simulink model "data_genrator"  (R2025b)
settings: Solver=FixedStepDiscrete  StartTime=0.0  StopTime=1800  FixedStep=2  RelTol=1e-3
libraries: instrumentseriallib x2
settings Model: Creator=Dell  LastModifiedBy=Dell

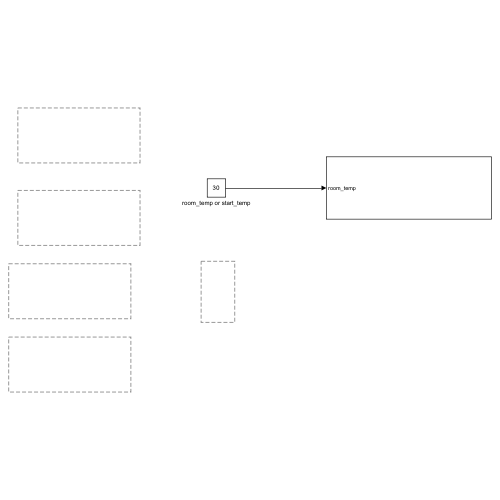
[thumbnail: Simulink's stored preview of the top-level diagram]
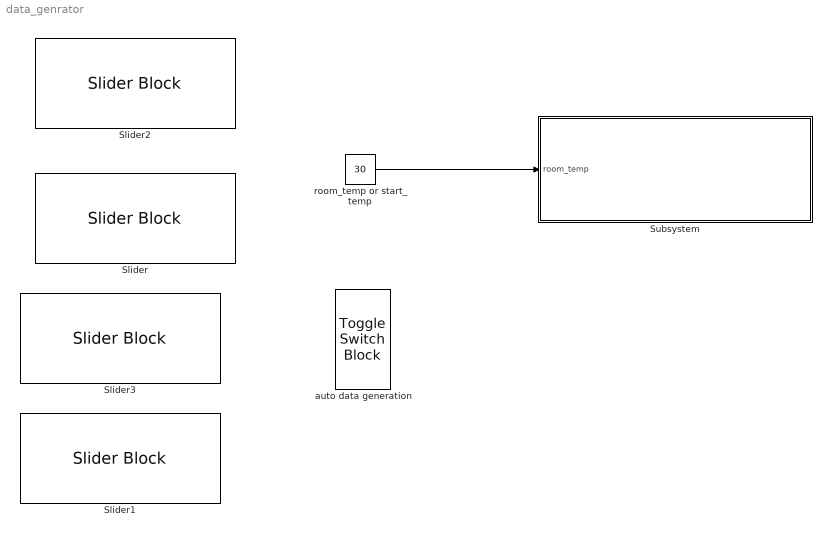
== system data_genrator ==
  Slider : SliderBlock
  Slider1 : SliderBlock  ScaleMax=2
  Slider2 : SliderBlock
  Slider3 : SliderBlock  ScaleMax=2
  Subsystem : Subsystem
  "auto data generation " : ToggleSwitchBlock
  room_temp or start_temp : Constant  Value=30
  wires:
  room_temp or start_temp/1 -> Subsystem/1(room_temp)

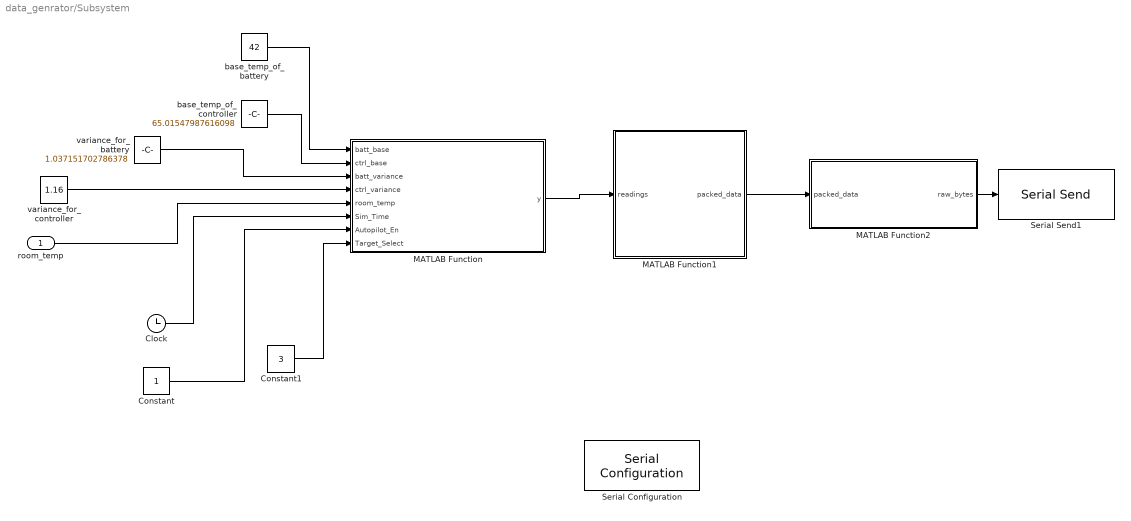
== system data_genrator/Subsystem ==
  room_temp : Inport
  Clock : Clock
  Constant : Constant
  Constant1 : Constant  Value=3
  MATLAB Function : MATLAB Function  TreatAsAtomicUnit=on
  MATLAB Function1 : MATLAB Function  TreatAsAtomicUnit=on
  MATLAB Function2 : MATLAB Function  TreatAsAtomicUnit=on
  Serial Configuration : instrumentseriallib/Serial Configuration  Priority=-200000  PortSel=COM8  Port=COM8  ComPort=COM8  BaudRate=115200  DataBits=8  Parity=none  StopBits=1  ByteOrder=little-endian  FlowControl=none  Timeout=10  SimulateUsing=Interpreted execution  BlockInModel=on  aMode=1
  Serial Send1 : instrumentseriallib/Serial Send  Priority=1  PortSel=COM8  Port=COM8  ComPort=COM8  Header=[]  Terminator=<none>  CustomTerminator=[]  EnableBlockingMode=on  SimulateUsing=Interpreted execution  BlockInModel=on  aMode=1
  base_temp_of_battery : Constant  Value=42
  base_temp_of_controller : Constant  Value=65.01547987616098
  variance_for_battery : Constant  Value=1.037151702786378
  variance_for_controller : Constant  Value=1.16
  wires:
  base_temp_of_controller/1 -> MATLAB Function/2(ctrl_base)
  variance_for_controller/1 -> MATLAB Function/4(ctrl_variance)
  base_temp_of_battery/1 -> MATLAB Function/1(batt_base)
  MATLAB Function2/1(raw_bytes) -> Serial Send1/1
  variance_for_battery/1 -> MATLAB Function/3(batt_variance)
  MATLAB Function1/1(packed_data) -> MATLAB Function2/1(packed_data)
  MATLAB Function/1(y) -> MATLAB Function1/1(readings)
  room_temp/1 -> MATLAB Function/5(room_temp)
  Clock/1 -> MATLAB Function/6(Sim_Time)
  Constant/1 -> MATLAB Function/7(Autopilot_En)
  Constant1/1 -> MATLAB Function/8(Target_Select)

== matlab function data_genrator/Subsystem/MATLAB Function1 ==
  data: readings input; packed_data output
function packed_data = Data_Organizer(readings)
    % readings: 16x1 vector of raw sensor values from sensor_simulator
    
    % Core hardware tracking addresses (16x1)
    addresses = [101:108, 201:208]'; 
    
    % Placeholders for the microcontroller to compute later (16x1)
    placeholder_average = zeros(16, 1);
    
    % Combine into a strict 16x3 matrix output
    packed_data = [addresses, readings, placeholder_average];
end

== matlab function data_genrator/Subsystem/MATLAB Function ==
  data: batt_base input; y output; ctrl_base input; batt_variance input; ctrl_variance input; room_temp input; Sim_Time input; Autopilot_En input; Target_Select input
function y = sensor_simulator_autopilot(batt_base, ctrl_base, batt_variance, ctrl_variance, room_temp, Sim_Time, Autopilot_En, Target_Select)
    % % Inputs:
    % batt_base: Target temp for battery (Slider 1)
    % ctrl_base: Target temp for controller (Slider 2)
    % batt_variance: Noise % for battery (Slider 3)
    % ctrl_variance: Noise % for controller (Slider 4)
    % room_temp: Starting ambient temperature from external constant block
    % Sim_Time: Continuous simulation Clock block input
    % Autopilot_En: Toggle switch (0 = Manual control, 1 = ML Data Generator)
    % Target_Select: Route fault variance (1 = Battery, 2 = Controller, 3 = Both)
    
    % --- 1. CORE THERMODYNAMIC BASELINE GENERATOR ---
    % Track internal thermal buildup over time
    persistent thermal_step;
    if isempty(thermal_step)
        thermal_step = 0;
    end
    
    % Increment time steps dynamically to simulate thermodynamic inertia
    thermal_step = thermal_step + 0.05; 
    warmup_factor = 1 - exp(-thermal_step);
    
    % Calculate the dynamic, rising core profiles based on dynamic room_temp
    current_batt_center = room_temp + (batt_base - room_temp) * warmup_factor;
    current_ctrl_center = room_temp + (ctrl_base - room_temp) * warmup_factor;
    
    % Convert the 0-100 slider inputs to decimal percentages
    dec_batt_var = batt_variance / 100;
    dec_ctrl_var = ctrl_variance / 100;
    
    % Generate 16 completely independent random factors between -1 and 1
    random_factors = (2 * rand(16, 1) - 1);
    
    % Initialize our output array
    y = zeros(16, 1);
    
    % Compute standard baseline profiles with scaled noise distribution offsets
    max_batt_offset = current_batt_center * dec_batt_var;
    y(1:8) = current_batt_center + (random_factors(1:8) * max_batt_offset);
    
    max_ctrl_offset = current_ctrl_center * dec_ctrl_var;
    y(9:16) = current_ctrl_center + (random_factors(9:16) * max_ctrl_offset);
    
    % ===================================================================
    % MODE ARBITRATION: IF AUTOPILOT IS OFF (0), EXIT HERE WITH MANUAL DATA
    % ===================================================================
    if Autopilot_En == 0
        return;
    end
    
    % ===================================================================
    % MODE ARBITRATION: IF AUTOPILOT IS ON (1), INJECT AUTOMATED VARIANCE
    % ===================================================================
    % Your slider profiles (warmup curve + noise) act as the active baseline.
    % The state machine superimposes automated operational trends over time.
    
    % Phase A: Seconds 0 to 60 -> Nominal Warmup Window
    if Sim_Time >= 0 && Sim_Time < 60
        % Let your baseline thermodynamic warmup factor dominate the curve naturally.
        % We just add a minor secondary cyclic operational ripple wave across all channels.
        for i = 1:16
            y(i) = y(i) + (0.3 * sin(Sim_Time * 2.5));
        end
        
    % Phase B: Seconds 60 to 180 -> Cyclic Load Transients (Stress Variance)
    elseif Sim_Time >= 60 && Sim_Time < 180
        elapsed_phase = Sim_Time - 60;
        % Generates a thermal fluctuation wave that slowly climbs
        thermal_wave = 4.0 * sin(elapsed_phase * 0.12) + (0.05 * elapsed_phase);
        for i = 1:16
            y(i) = y(i) + thermal_wave;
        end
        
    % Phase C: Seconds 180 Onwards -> Accelerated Failure Curve (ML Target Data)
    elseif Sim_Time >= 180
        elapsed_runaway = Sim_Time - 180;
        % Exponential growth profile to provide predictable degradation data points
        runaway_slope = 1.15 * (elapsed_runaway ^ 1.16);
        
        % Read Target_Select to inject the anomaly variance into the correct index
        if Target_Select == 1
            % Inject exclusively into Battery Pack Module Cell 04 (Index 4 / Sensor ID 104)
            y(4) = y(4) + runaway_slope;
            
        elseif Target_Select == 2
            % Inject exclusively into Inverter Controller Layer 04 (Index 12 / Sensor ID 204)
            y(12) = y(12) + runaway_slope;
            
        elseif Target_Select == 3
            % Parallel Overload: Inject into both subsystems simultaneously (Indices 4 and 12)
            y(4) = y(4) + runaway_slope;
            y(12) = y(12) + runaway_slope;
        end
    end
end

== matlab function data_genrator/Subsystem/MATLAB Function2 ==
  data: packed_data input; raw_bytes output
function raw_bytes = Serial_Telemetry(packed_data)
    % packed_data: 16x3 matrix input from Data_Organizer
    
    % 1. Preallocate a strictly fixed-size character buffer (200 bytes)
    buf = char(32 * ones(1, 200)); % Fills buffer with trailing spaces (ASCII 32)
    ptr = 1;
    
    for i = 1:16
        % FIX: Convert address to int16 (signed) instead of uint16 to match '%03d'
        addr = int16(packed_data(i, 1));
        val = packed_data(i, 2);
        
        % %03d forces a 3-digit sensor address string (e.g., 101)
        % %06.2f forces an exact 6-character floating temperature width (e.g., 032.45)
        entry_str = sprintf('%03d:%06.2f,', addr, val);
        
        % Drop the formatted text chunk directly into its pre-allocated slot
        buf(ptr : ptr + 10) = entry_str;
        ptr = ptr + 11;
    end
    
    % 2. Place an explicit frame-termination line-break at the data boundary end
    buf(ptr) = char(10); % ASCII 10 maps directly to '\n'
    
    % 3. Output the finalized byte structure as a fixed-dimension vector
    raw_bytes = uint8(buf)';
end
